simulink model "FinSimLagrange1"  (R2020b)
settings: Solver=FixedStepAuto  StartTime=0.0  StopTime=10.0  FixedStep=0.001  RelTol=1e-3
values from neighbouring files (symbols this model uses):
  m = {0 0 0 0 0}    [DynMatrixCalculator.m]    (also in DynMats_Iterative.mat = ; FinLagrange_2.m = mass{i})
  N = {zeros(3,1) zeros(3,1) zeros(3,1) zeros(3,1) zeros(3,1)}    [DynMatrixCalculator.m]    (also in DynMats_Iterative.mat = )
undefined symbols (not defined in the file or in its folder): X, Y, Z
libraries: sm_lib x34, nesl_utility x24
(part 2 of 4)

== matlab function FinSimLagrange1/Tau Lagrange/MATLAB Function ==
  data: theta input; theta_d input; theta_2d input; Force output; tau2 output; tau3 output; tau4 output
function [Force, tau2, tau3, tau4] = fcn(theta, theta_d, theta_2d)

q1 = theta(1);    q_d1 = theta_d(1);
q2 = theta(2);    q_d2 = theta_d(2);
q3 = theta(3);    q_d3 = theta_d(3);
q4 = theta(4);    q_d4 = theta_d(4);

%% M
M= [                                                                                                                                                                                                                                                                                                                                                                                                                                            27947/500,                                                                                                                                                                                                                                                                                                                                                                                                                                                                                                                                                                                                                                                                                                                                                                                                             (252799*cos(q2))/4000000 + (8197271897754683*sin(q2))/576460752303423488 + (5271805637408845*cos(q2)*cos(q3))/36028797018963968 + (65855377368601641551*cos(q2)*sin(q3))/14073748835532800000 - (6905770129014017*cos(q2)*cos(q3)*cos(q4))/4503599627370496 + (1448762964128815*cos(q2)*cos(q3)*sin(q4))/9007199254740992 + (1448762964128815*cos(q2)*cos(q4)*sin(q3))/9007199254740992 + (6905770129014017*cos(q2)*sin(q3)*sin(q4))/4503599627370496,                                                                                                                                                                  (sin(q2)*(18109537051610187500*cos(q3 + q4) + 172644253225350425000*sin(q3 + q4) + 526843018948813132408*cos(q3) - 16474392616902640625*sin(q3)))/112589990684262400000,                                          (sin(q2)*(1448762964128815*cos(q3 + q4) + 13811540258028034*sin(q3 + q4)))/9007199254740992
(252799*cos(q2))/4000000 + (8197271897754683*sin(q2))/576460752303423488 + (5271805637408845*cos(q2)*cos(q3))/36028797018963968 + (65855377368601641551*cos(q2)*sin(q3))/14073748835532800000 - (6905770129014017*cos(q2)*cos(q3)*cos(q4))/4503599627370496 + (1448762964128815*cos(q2)*cos(q3)*sin(q4))/9007199254740992 + (1448762964128815*cos(q2)*cos(q4)*sin(q3))/9007199254740992 + (6905770129014017*cos(q2)*sin(q3)*sin(q4))/4503599627370496, (62207306521424371*cos(q3))/360287970189639680000 - (8070931876976101*sin(2*q4))/576460752303423488 - (16294718663493729*sin(2*q3))/576460752303423488 + (8402825191947127*cos(q4))/90071992547409920 + (3885467264747496851509*sin(q3))/703687441776640000000000 + (200267333741406493*sin(q4))/225179981368524800 - (407440437611827003*cos(q3)*cos(q4))/225179981368524800000 + (17095402976720017*cos(q3)*sin(q4))/90071992547409920000 + (17095402976720017*cos(q4)*sin(q3))/90071992547409920000 + (407440437611827003*sin(q3)*sin(q4))/225179981368524800000 - (1109907735748447107177*cos(q3)^2)/703687441776640000000 - (6572768604275487*cos(q4)^2)/18014398509481984 - (8402825191947127*cos(q3)^2*cos(q4))/90071992547409920 - (200267333741406493*cos(q3)^2*sin(q4))/225179981368524800 + (6572768604275487*cos(q3)^2*cos(q4)^2)/9007199254740992 + (8070931876976101*cos(q3)*cos(q4)^2*sin(q3))/144115188075855872 + (8070931876976101*cos(q3)^2*cos(q4)*sin(q4))/144115188075855872 - (200267333741406493*cos(q3)*cos(q4)*sin(q3))/225179981368524800 + (8402825191947127*cos(q3)*sin(q3)*sin(q4))/90071992547409920 - (6572768604275487*cos(q3)*cos(q4)*sin(q3)*sin(q4))/9007199254740992 + 24003950885205506270535387/14073748835532800000000000, (31130840590942719*cos(q3))/57646075230342348800 + (5398328972706657*sin(q3))/36893488147419103232 - (2967066550535813*cos(q3)*cos(q4))/18446744073709551616 - (1229911296841483*cos(q3)*sin(q4))/2305843009213693952 - (1229911296841483*cos(q4)*sin(q3))/2305843009213693952 + (2967066550535813*sin(q3)*sin(q4))/18446744073709551616,               -(105615118993599592856087292485465^(1/2)*cos(q3 + q4 - atan(9839290374731864/2967066550535813)))/18446744073709551616
                                                                                                                                                                                                                                                                              (sin(q2)*(18109537051610187500*cos(q3 + q4) + 172644253225350425000*sin(q3 + q4) + 526843018948813132408*cos(q3) - 16474392616902640625*sin(q3)))/112589990684262400000,                                                                                                                                                                                                                                                                                                                                                                                                                                                                                                                                                                                                                                                                                                                                                                                                                                                                                                                          (31130840590942719*cos(q3))/57646075230342348800 + (5398328972706657*sin(q3))/36893488147419103232 - (2967066550535813*cos(q3)*cos(q4))/18446744073709551616 - (1229911296841483*cos(q3)*sin(q4))/2305843009213693952 - (1229911296841483*cos(q4)*sin(q3))/2305843009213693952 + (2967066550535813*sin(q3)*sin(q4))/18446744073709551616,                                                                                                                                                                                             (8402825191947127*cos(q4))/90071992547409920 + (200267333741406493*sin(q4))/225179981368524800 + 286280843871266757263/175921860444160000000, (8402825191947127*cos(q4))/180143985094819840 + (200267333741406493*sin(q4))/450359962737049600 + 6947924758274927/18014398509481984
                                                                                                                                                                                                                                                                                                                                                          (sin(q2)*(1448762964128815*cos(q3 + q4) + 13811540258028034*sin(q3 + q4)))/9007199254740992,                                                                                                                                                                                                                                                                                                                                                                                                                                                                                                                                                                                                                                                                                                                                                                                                                                                                                                                                                                                                                                                                                                                                            -(105615118993599592856087292485465^(1/2)*cos(q3 + q4 - atan(9839290374731864/2967066550535813)))/18446744073709551616,                                                                                                                                                                                                     (8402825191947127*cos(q4))/180143985094819840 + (200267333741406493*sin(q4))/450359962737049600 + 6947924758274927/18014398509481984,                                                                                                   6947924758274927/18014398509481984];

%% V
V=[                                                                                                                                                                                                                                                                                                                                                                                                                                                                                                                                                                                                                                                                                                                                                                                                                                                                                                                                                                                                                                                                                                                                                                                          0,                                                                                                                                                                                                                                                                                                                                                                                                                                                                                                                                                                                                                                                                                                                                                                                                                                                                                                                                                                                (q_d4*cos(q2)*(1448762964128815*cos(q3 + q4) + 13811540258028034*sin(q3 + q4)))/9007199254740992 - q_d2*((252799*sin(q2))/4000000 - (8197271897754683*cos(q2))/576460752303423488 + (5271805637408845*cos(q3)*sin(q2))/36028797018963968 + (65855377368601641551*sin(q2)*sin(q3))/14073748835532800000 + (6905770129014017*sin(q2)*sin(q3)*sin(q4))/4503599627370496 - (6905770129014017*cos(q3)*cos(q4)*sin(q2))/4503599627370496 + (1448762964128815*cos(q3)*sin(q2)*sin(q4))/9007199254740992 + (1448762964128815*cos(q4)*sin(q2)*sin(q3))/9007199254740992) + (q_d3*cos(q2)*(18109537051610187500*cos(q3 + q4) + 172644253225350425000*sin(q3 + q4) + 526843018948813132408*cos(q3) - 16474392616902640625*sin(q3)))/112589990684262400000,                                                                                                                                                                                                                                                                                                 (q_d2*cos(q2)*(18109537051610187500*cos(q3 + q4) + 172644253225350425000*sin(q3 + q4) + 526843018948813132408*cos(q3) - 16474392616902640625*sin(q3)))/112589990684262400000 - (q_d3*sin(q2)*(18109537051610187500*sin(q3 + q4) - 172644253225350425000*cos(q3 + q4) + 16474392616902640625*cos(q3) + 526843018948813132408*sin(q3)))/112589990684262400000 + (q_d4*sin(q2)*(172644253225350425000*cos(q3 + q4) - 18109537051610187500*sin(q3 + q4)))/112589990684262400000,                                                      (q_d2*cos(q2)*(1448762964128815*cos(q3 + q4) + 13811540258028034*sin(q3 + q4)))/9007199254740992 + (q_d3*sin(q2)*(13811540258028034*cos(q3 + q4) - 1448762964128815*sin(q3 + q4)))/9007199254740992 + (q_d4*sin(q2)*(13811540258028034*cos(q3 + q4) - 1448762964128815*sin(q3 + q4)))/9007199254740992
(8197271897754683*q_d2*cos(q2))/1152921504606846976 - (252799*q_d2*sin(q2))/8000000 + (65855377368601641551*q_d3*cos(q2)*cos(q3))/28147497671065600000 - (5271805637408845*q_d2*cos(q3)*sin(q2))/72057594037927936 - (5271805637408845*q_d3*cos(q2)*sin(q3))/72057594037927936 - (65855377368601641551*q_d2*sin(q2)*sin(q3))/28147497671065600000 + (1448762964128815*q_d3*cos(q2)*cos(q3)*cos(q4))/18014398509481984 + (1448762964128815*q_d4*cos(q2)*cos(q3)*cos(q4))/18014398509481984 + (6905770129014017*q_d2*cos(q3)*cos(q4)*sin(q2))/9007199254740992 + (6905770129014017*q_d3*cos(q2)*cos(q3)*sin(q4))/9007199254740992 + (6905770129014017*q_d3*cos(q2)*cos(q4)*sin(q3))/9007199254740992 + (6905770129014017*q_d4*cos(q2)*cos(q3)*sin(q4))/9007199254740992 + (6905770129014017*q_d4*cos(q2)*cos(q4)*sin(q3))/9007199254740992 - (1448762964128815*q_d2*cos(q3)*sin(q2)*sin(q4))/18014398509481984 - (1448762964128815*q_d2*cos(q4)*sin(q2)*sin(q3))/18014398509481984 - (1448762964128815*q_d3*cos(q2)*sin(q3)*sin(q4))/18014398509481984 - (1448762964128815*q_d4*cos(q2)*sin(q3)*sin(q4))/18014398509481984 - (6905770129014017*q_d2*sin(q2)*sin(q3)*sin(q4))/9007199254740992, (1706317924287871792479*q_d3*sin(2*q3))/1407374883553280000000 - (2055946696629407*q_d3*cos(2*q3))/72057594037927936 + (8070931876976101*q_d3*cos(2*q3 + 2*q4))/288230376151711744 + (8070931876976101*q_d4*cos(2*q3 + 2*q4))/288230376151711744 - (6572768604275487*q_d3*sin(2*q3 + 2*q4))/18014398509481984 - (6572768604275487*q_d4*sin(2*q3 + 2*q4))/18014398509481984 + (1448762964128815*q_d1*cos(q3 - q2 + q4))/36028797018963968 + (6905770129014017*q_d1*sin(q3 - q2 + q4))/18014398509481984 - (65855377368601641551*q_d1*cos(q2 + q3))/56294995342131200000 + (17095402976720017*q_d3*cos(q3 + q4))/90071992547409920000 + (17095402976720017*q_d4*cos(q3 + q4))/90071992547409920000 + (5271805637408845*q_d1*sin(q2 + q3))/144115188075855872 + (407440437611827003*q_d3*sin(q3 + q4))/225179981368524800000 + (407440437611827003*q_d4*sin(q3 + q4))/225179981368524800000 - (8197271897754683*q_d1*cos(q2))/1152921504606846976 + (3885467264747496851509*q_d3*cos(q3))/703687441776640000000000 + (200267333741406493*q_d4*cos(q4))/450359962737049600 + (252799*q_d1*sin(q2))/8000000 - (62207306521424371*q_d3*sin(q3))/360287970189639680000 - (8402825191947127*q_d4*sin(q4))/180143985094819840 + (65855377368601641551*q_d1*cos(q2 - q3))/56294995342131200000 - (200267333741406493*q_d3*cos(2*q3 + q4))/225179981368524800 - (200267333741406493*q_d4*cos(2*q3 + q4))/450359962737049600 + (5271805637408845*q_d1*sin(q2 - q3))/144115188075855872 + (8402825191947127*q_d3*sin(2*q3 + q4))/90071992547409920 + (8402825191947127*q_d4*sin(2*q3 + q4))/180143985094819840 - (1448762964128815*q_d1*cos(q2 + q3 + q4))/36028797018963968 - (6905770129014017*q_d1*sin(q2 + q3 + q4))/18014398509481984, q_d3*((5398328972706657*cos(q3))/36893488147419103232 - (31130840590942719*sin(q3))/57646075230342348800 - (1229911296841483*cos(q3)*cos(q4))/2305843009213693952 + (2967066550535813*cos(q3)*sin(q4))/18446744073709551616 + (2967066550535813*cos(q4)*sin(q3))/18446744073709551616 + (1229911296841483*sin(q3)*sin(q4))/2305843009213693952) + q_d4*((2967066550535813*cos(q3)*sin(q4))/18446744073709551616 - (1229911296841483*cos(q3)*cos(q4))/2305843009213693952 + (2967066550535813*cos(q4)*sin(q3))/18446744073709551616 + (1229911296841483*sin(q3)*sin(q4))/2305843009213693952) - (q_d1*cos(q2)*(18109537051610187500*cos(q3 + q4) + 172644253225350425000*sin(q3 + q4) + 526843018948813132408*cos(q3) - 16474392616902640625*sin(q3)))/225179981368524800000, (105615118993599592856087292485465^(1/2)*q_d3*sin(q3 + q4 - atan(9839290374731864/2967066550535813)))/18446744073709551616 - (q_d1*cos(q2)*(1448762964128815*cos(q3 + q4) + 13811540258028034*sin(q3 + q4)))/18014398509481984 + (105615118993599592856087292485465^(1/2)*q_d4*sin(q3 + q4 - atan(9839290374731864/2967066550535813)))/18446744073709551616
                                                                                                                                                                                                                                                (1448762964128815*q_d2*cos(q3 + q4)*cos(q2))/9007199254740992 + (6905770129014017*q_d2*sin(q3 + q4)*cos(q2))/4503599627370496 + (6905770129014017*q_d3*cos(q3 + q4)*sin(q2))/9007199254740992 + (6905770129014017*q_d4*cos(q3 + q4)*sin(q2))/9007199254740992 - (1448762964128815*q_d3*sin(q3 + q4)*sin(q2))/18014398509481984 - (1448762964128815*q_d4*sin(q3 + q4)*sin(q2))/18014398509481984 + (65855377368601641551*q_d2*cos(q2)*cos(q3))/28147497671065600000 - (5271805637408845*q_d2*cos(q2)*sin(q3))/72057594037927936 - (5271805637408845*q_d3*cos(q3)*sin(q2))/72057594037927936 - (65855377368601641551*q_d3*sin(q2)*sin(q3))/28147497671065600000 - (1448762964128815*q_d2*cos(q2)*cos(q3)*cos(q4))/18014398509481984 - (6905770129014017*q_d2*cos(q2)*cos(q3)*sin(q4))/9007199254740992 - (6905770129014017*q_d2*cos(q2)*cos(q4)*sin(q3))/9007199254740992 + (1448762964128815*q_d2*cos(q2)*sin(q3)*sin(q4))/18014398509481984,                                                                                                                                                                                                                  (2055946696629407*q_d2*cos(2*q3))/144115188075855872 - (1706317924287871792479*q_d2*sin(2*q3))/2814749767106560000000 - (8070931876976101*q_d2*cos(2*q3 + 2*q4))/576460752303423488 + (6572768604275487*q_d2*sin(2*q3 + 2*q4))/36028797018963968 - (1448762964128815*q_d1*cos(q3 - q2 + q4))/36028797018963968 - (6905770129014017*q_d1*sin(q3 - q2 + q4))/18014398509481984 - (65855377368601641551*q_d1*cos(q2 + q3))/56294995342131200000 - (17095402976720017*q_d2*cos(q3 + q4))/180143985094819840000 - (1229911296841483*q_d3*cos(q3 + q4))/4611686018427387904 - (1229911296841483*q_d4*cos(q3 + q4))/4611686018427387904 + (5271805637408845*q_d1*sin(q2 + q3))/144115188075855872 - (407440437611827003*q_d2*sin(q3 + q4))/450359962737049600000 + (2967066550535813*q_d3*sin(q3 + q4))/36893488147419103232 + (2967066550535813*q_d4*sin(q3 + q4))/36893488147419103232 - (3885467264747496851509*q_d2*cos(q3))/1407374883553280000000000 + (5398328972706657*q_d3*cos(q3))/73786976294838206464 + (62207306521424371*q_d2*sin(q3))/720575940379279360000 - (31130840590942719*q_d3*sin(q3))/115292150460684697600 - (65855377368601641551*q_d1*cos(q2 - q3))/56294995342131200000 + (200267333741406493*q_d2*cos(2*q3 + q4))/450359962737049600 - (5271805637408845*q_d1*sin(q2 - q3))/144115188075855872 - (8402825191947127*q_d2*sin(2*q3 + q4))/180143985094819840 - (1448762964128815*q_d1*cos(q2 + q3 + q4))/36028797018963968 - (6905770129014017*q_d1*sin(q2 + q3 + q4))/18014398509481984,                                                                                                                                  q_d4*((200267333741406493*cos(q4))/225179981368524800 - (8402825191947127*sin(q4))/90071992547409920) - (q_d2*((5398328972706657*cos(q3))/36893488147419103232 - (31130840590942719*sin(q3))/57646075230342348800 - (1229911296841483*cos(q3)*cos(q4))/2305843009213693952 + (2967066550535813*cos(q3)*sin(q4))/18446744073709551616 + (2967066550535813*cos(q4)*sin(q3))/18446744073709551616 + (1229911296841483*sin(q3)*sin(q4))/2305843009213693952))/2 + (q_d1*sin(q2)*(18109537051610187500*sin(q3 + q4) - 172644253225350425000*cos(q3 + q4) + 16474392616902640625*cos(q3) + 526843018948813132408*sin(q3)))/225179981368524800000,                     q_d4*((200267333741406493*cos(q4))/450359962737049600 - (8402825191947127*sin(q4))/180143985094819840) - (105615118993599592856087292485465^(1/2)*q_d2*sin(q3 + q4 - atan(9839290374731864/2967066550535813)))/36893488147419103232 - (q_d1*sin(q2)*(13811540258028034*cos(q3 + q4) - 1448762964128815*sin(q3 + q4)))/18014398509481984
                                                                                                                                                                                                                                                                                                                                                                                                                                                                                                              (1448762964128815*q_d2*cos(q3 + q4)*cos(q2))/9007199254740992 + (6905770129014017*q_d2*sin(q3 + q4)*cos(q2))/4503599627370496 + (6905770129014017*q_d3*cos(q3 + q4)*sin(q2))/9007199254740992 + (6905770129014017*q_d4*cos(q3 + q4)*sin(q2))/9007199254740992 - (1448762964128815*q_d3*sin(q3 + q4)*sin(q2))/18014398509481984 - (1448762964128815*q_d4*sin(q3 + q4)*sin(q2))/18014398509481984 - (1448762964128815*q_d2*cos(q2)*cos(q3)*cos(q4))/18014398509481984 - (6905770129014017*q_d2*cos(q2)*cos(q3)*sin(q4))/9007199254740992 - (6905770129014017*q_d2*cos(q2)*cos(q4)*sin(q3))/9007199254740992 + (1448762964128815*q_d2*cos(q2)*sin(q3)*sin(q4))/18014398509481984,                                                                                                                                                                                                                                                                                                                                                                                                                                                                                                                                                                                                                                                                                                                             (6572768604275487*q_d2*sin(2*q3 + 2*q4))/36028797018963968 - (8070931876976101*q_d2*cos(2*q3 + 2*q4))/576460752303423488 - (1448762964128815*q_d1*cos(q3 - q2 + q4))/36028797018963968 - (6905770129014017*q_d1*sin(q3 - q2 + q4))/18014398509481984 - (17095402976720017*q_d2*cos(q3 + q4))/180143985094819840000 - (1229911296841483*q_d3*cos(q3 + q4))/4611686018427387904 - (1229911296841483*q_d4*cos(q3 + q4))/4611686018427387904 - (407440437611827003*q_d2*sin(q3 + q4))/450359962737049600000 + (2967066550535813*q_d3*sin(q3 + q4))/36893488147419103232 + (2967066550535813*q_d4*sin(q3 + q4))/36893488147419103232 - (200267333741406493*q_d2*cos(q4))/900719925474099200 + (8402825191947127*q_d2*sin(q4))/360287970189639680 + (200267333741406493*q_d2*cos(2*q3 + q4))/900719925474099200 - (8402825191947127*q_d2*sin(2*q3 + q4))/360287970189639680 - (1448762964128815*q_d1*cos(q2 + q3 + q4))/36028797018963968 - (6905770129014017*q_d1*sin(q2 + q3 + q4))/18014398509481984,                                                                                                                                                                                     (q_d4*((200267333741406493*cos(q4))/450359962737049600 - (8402825191947127*sin(q4))/180143985094819840))/2 - (q_d3*((200267333741406493*cos(q4))/225179981368524800 - (8402825191947127*sin(q4))/90071992547409920))/2 - (q_d2*((2967066550535813*cos(q3)*sin(q4))/18446744073709551616 - (1229911296841483*cos(q3)*cos(q4))/2305843009213693952 + (2967066550535813*cos(q4)*sin(q3))/18446744073709551616 + (1229911296841483*sin(q3)*sin(q4))/2305843009213693952))/2 - (q_d1*sin(q2)*(172644253225350425000*cos(q3 + q4) - 18109537051610187500*sin(q3 + q4)))/225179981368524800000,                                       (105615118993599592856087292485465^(1/2)*q_d2*cos(q3 + q4 + atan(2967066550535813/9839290374731864)))/36893488147419103232 - (q_d1*sin(q2)*(13811540258028034*cos(q3 + q4) - 1448762964128815*sin(q3 + q4)))/18014398509481984 - (29*q_d3*(13811540258028034*cos(q4) - 1448762964128815*sin(q4)))/1801439850948198400];

%% G
G=[                                                                                                                                                                                                                                                                                                                                                    0
                                                                                                                                                                                                                                                                                                                                                    0
(6774560496562750677*cos(q3)*cos(q4))/450359962737049600 - (64604125198598210361531*sin(q3))/1407374883553280000000 - (1034328266059615389*cos(q3))/720575940379279360 - (284247293562073503*cos(q3)*sin(q4))/180143985094819840 - (284247293562073503*cos(q4)*sin(q3))/180143985094819840 - (6774560496562750677*sin(q3)*sin(q4))/450359962737049600
                                                                                                                                                                                                                             (981*192857558425360402101618243209381^(1/2)*cos(q3 + q4 + atan(1448762964128815/13811540258028034)))/900719925474099200];

%% Tau
Tau = M*theta_2d + V*theta_d + G;
Force=Tau(1); tau2=Tau(2); tau3=Tau(3); tau4=Tau(4);

== matlab function FinSimLagrange1/MATLAB Function ==
  data: t input; theta output size=[4,1]
function theta = fcn(t)

theta = [0;0;0;0];

theta(1) = sin(t);
theta(2) = sin(t);
theta(3) = sin(t);
theta(4) = sin(t);

== matlab function FinSimLagrange1/End Effector/MATLAB Function ==
  data: theta input; theta_d input; theta_2d input; EndEffector output
function EndEffector = fcn1(theta, theta_d, theta_2d)

q1 = theta(1);    q_d1 = theta_d(1);
q2 = theta(2);    q_d2 = theta_d(2);
q3 = theta(3);    q_d3 = theta_d(3);
q4 = theta(4);    q_d4 = theta_d(4);

%% T
T = zeros(4,4,5);

T(:,:,1) = [1,0,0,0 ; 0,1,0,0 ; 0,0,1,q1 ; 0,0,0,1];


T(:,:,2) = [ cos(q2), -sin(q2), 0,        0
       0,        0, 1, 197/1000
-sin(q2), -cos(q2), 0,       q1
       0,        0, 0,        1];


T(:,:,3) = [-cos(q2)*sin(q3), -cos(q2)*cos(q3), sin(q2),     -(59*cos(q2))/100000
         cos(q3),         -sin(q3),       0,                 873/2500
 sin(q2)*sin(q3),  cos(q3)*sin(q2), cos(q2), q1 + (59*sin(q2))/100000
               0,                0,       0,                        1];


T(:,:,4) = [cos(q2)*cos(q3)*cos(q4) - cos(q2)*sin(q3)*sin(q4), - cos(q2)*cos(q3)*sin(q4) - cos(q2)*cos(q4)*sin(q3), sin(q2),    - (59*cos(q2))/100000 - (29*cos(q2)*sin(q3))/100
                cos(q3)*sin(q4) + cos(q4)*sin(q3),                   cos(q3)*cos(q4) - sin(q3)*sin(q4),       0,                         (29*cos(q3))/100 + 873/2500
sin(q2)*sin(q3)*sin(q4) - cos(q3)*cos(q4)*sin(q2),   cos(q3)*sin(q2)*sin(q4) + cos(q4)*sin(q2)*sin(q3), cos(q2), q1 + (59*sin(q2))/100000 + (29*sin(q2)*sin(q3))/100
                                                0,                                                   0,       0,                                                   1];


T(:,:,5) = [cos(q2)*cos(q3)*cos(q4) - cos(q2)*sin(q3)*sin(q4), - cos(q2)*cos(q3)*sin(q4) - cos(q2)*cos(q4)*sin(q3), sin(q2),      (1913*cos(q2)*cos(q3)*cos(q4))/5000 - (29*cos(q2)*sin(q3))/100 - (59*cos(q2))/100000 - (cos(q2)*cos(q3)*sin(q4))/50 - (cos(q2)*cos(q4)*sin(q3))/50 - (1913*cos(q2)*sin(q3)*sin(q4))/5000
                cos(q3)*sin(q4) + cos(q4)*sin(q3),                   cos(q3)*cos(q4) - sin(q3)*sin(q4),       0,                                                         (29*cos(q3))/100 + (cos(q3)*cos(q4))/50 + (1913*cos(q3)*sin(q4))/5000 + (1913*cos(q4)*sin(q3))/5000 - (sin(q3)*sin(q4))/50 + 873/2500
sin(q2)*sin(q3)*sin(q4) - cos(q3)*cos(q4)*sin(q2),   cos(q3)*sin(q2)*sin(q4) + cos(q4)*sin(q2)*sin(q3), cos(q2), q1 + (59*sin(q2))/100000 + (29*sin(q2)*sin(q3))/100 + (1913*sin(q2)*sin(q3)*sin(q4))/5000 - (1913*cos(q3)*cos(q4)*sin(q2))/5000 + (cos(q3)*sin(q2)*sin(q4))/50 + (cos(q4)*sin(q2)*sin(q3))/50
                                                0,                                                   0,       0,                                                                                                                                                                                             1];


%% P_end
EndEffector = T(1:3,4,end);
